simulink model "KugleArmTest1"  (R2018b)
settings: Solver=VariableStepAuto  StartTime=0.0  StopTime=100  RelTol=1e-3
libraries: vrlib x2, simulink x1, aerolibanimutils x1
settings Model: Creator=Yahya  LastModifiedBy=martinandersen

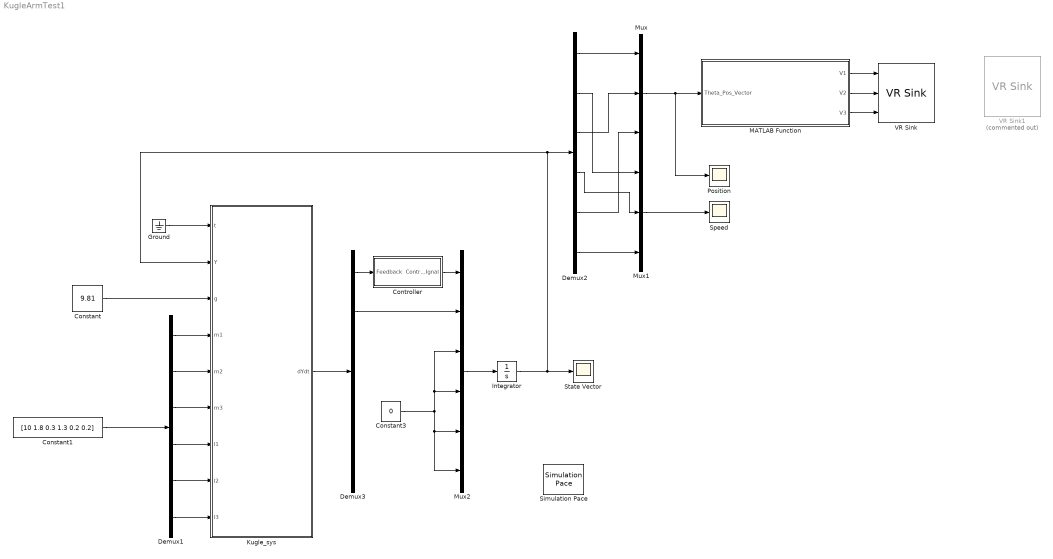
== system KugleArmTest1 ==
  Constant : Constant  Value=9.81
  Constant1 : Constant  Value=[10 1.8 0.3 1.3 0.2 0.2]
  Constant3 : Constant  Value=0
  Controller : Subsystem
  Demux1 : Demux  Outputs=6
  Demux2 : Demux  Outputs=6
  Demux3 : Demux  Outputs=6
  Ground : Ground
  Integrator : Integrator  InitialCondition=[1 0 90 0 45 0]*pi/180
  Kugle_sys : MATLAB Function  TreatAsAtomicUnit=on
  MATLAB Function : MATLAB Function  TreatAsAtomicUnit=on
  Mux : Mux  Inputs=3
  Mux1 : Mux  Inputs=3
  Mux2 : Mux  Inputs=6
  Position : Scope
  Simulation Pace : aerolibanimutils/Simulation Pace  SimulationPace=1  SleepMode=MATLAB Thread  OutputPaceError=off  SampleTime=1/30
      settings: AttributesFormatString=%<SimulationPace> sec/sec
  Speed : Scope
  State Vector : Scope
  VR Sink : vrlib/VR Sink  InstantiateOnLoad=on  SampleTime=0.1  ViewEnable=on  RemoteChange=off  RemoteView=off  FieldsWritten=JOINT_1.rotation.4.1.1.double#JOINT_2.rotation.4.1.1.double#JOINT_3.rotation.4.1.1.double  WorldFileName=Pendel3D1.wrl  AutoView=off  VideoDimensions=[]  AllowVariableSize=off  FigureProperties="{'Position', 'Name', 'Viewpoint', 'CameraBound', 'CameraDirection', 'CameraPosition', 'CameraUpVector', 'ZoomFactor', 'Antialiasing', 'Headlight', 'Lighting', 'NavPanel', 'Sound', 'StatusBar', 'Stereo3D', 'Stereo3DCameraOffset', 'Stereo3DHIT', 'ToolBar', 'Textures', 'Transparency', 'Triad', 'Wireframe', 'NavZones', 'NavMode', 'NavSpeed', 'CaptureFileFormat', 'CaptureFileName', 'Record2DCompressMethod', 'Record2DCompressQuality', 'Record2D', 'Record2DFileName', 'Record2DFPS'; [5.0000000000000000e+00   9.4000000000000000e+01   5.7600000000000000e+02   3.5000000000000000e+02], '', '', 'on', [0.0000000000000000e+00   0.0000000000000000e+00  -1.0000000000000000e+00], [0.0000000000000000e+00   0.0000000000000000e+00   1.0000000000000000e+01], [0.0000000000000000e+00   1.0000000000000000e+00   0.0000000000000000e+00], [1.0000000000000000e+00], 'on', 'on', 'on', 'halfbar', 'on', 'on', 'off', [1.0000000149011612e-01], [0.0000000000000000e+00], 'on', 'on', 'on', 'none', 'off', 'off', 'fly', 'normal', 'tif', '%f_anim_%n.tif', 'auto', [7.5000000000000000e+01], 'off', '%f_anim_%n.avi', 'auto'}"
      settings: SourceProductBaseCode=VR
  VR Sink1 : vrlib/VR Sink  Commented=on  InstantiateOnLoad=on  SampleTime=0.1  ViewEnable=on  RemoteChange=off  RemoteView=off  FieldsWritten=JOINT_1.rotation.4.1.1.double#JOINT_2.rotation.4.1.1.double#JOINT_3.rotation.4.1.1.double  WorldFileName=Pendel3D1.wrl  AutoView=off  VideoDimensions=[]  AllowVariableSize=off
      settings: SourceProductBaseCode=VR
  wires:
  Constant/1 -> Kugle_sys/3(g)
  Integrator/1 -> Kugle_sys/2(Y), Demux2/1, State Vector/1
  Ground/1 -> Kugle_sys/1(t)
  Demux1/1 -> Kugle_sys/4(m1)
  Demux1/2 -> Kugle_sys/5(m2)
  Demux1/3 -> Kugle_sys/6(m3)
  Demux1/4 -> Kugle_sys/7(l1)
  Demux1/5 -> Kugle_sys/8(l2)
  Demux1/6 -> Kugle_sys/9(l3)
  Constant1/1 -> Demux1/1
  Demux2/1 -> Mux/1
  Mux/1 -> MATLAB Function/1(Theta_Pos_Vector), Position/1
  Mux1/1 -> Speed/1
  Demux2/3 -> Mux/2
  Demux2/5 -> Mux/3
  Demux2/2 -> Mux1/1
  Demux2/4 -> Mux1/2
  Demux2/6 -> Mux1/3
  MATLAB Function/1(V1) -> VR Sink/1
  MATLAB Function/2(V2) -> VR Sink/2
  MATLAB Function/3(V3) -> VR Sink/3
  Kugle_sys/1(dYdt) -> Demux3/1
  Mux2/1 -> Integrator/1
  Constant3/1 -> Mux2/4, Mux2/3, Mux2/6, Mux2/5
  Demux3/2 -> Mux2/2
  Demux3/1 -> Controller/1(Feedback)
  Controller/1(Control SIgnal) -> Mux2/1

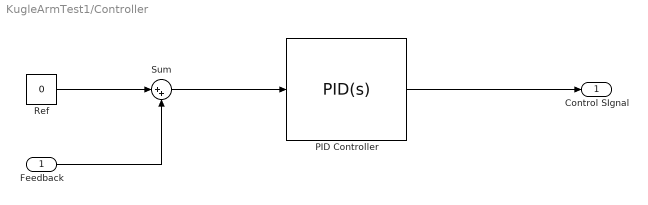
== system KugleArmTest1/Controller ==
  Feedback : Inport
  PID Controller : simulink/Continuous/PID Controller  Controller=PID  Form=Parallel  TimeDomain=Continuous-time  SampleTime=-1  IntegratorMethod=Forward Euler  FilterMethod=Forward Euler  ControllerParametersSource=internal  P=-0.0250583330761755  I=-0.00117310030702187  D=0  UseFilter=on  N=5.45397025421619  TunerSelectOption=Transfer Function Based (PID Tuner App)  InitialConditionSource=internal  InitialConditionForIntegrator=0  InitialConditionForFilter=0  DifferentiatorICPrevScaledInput=0  ExternalReset=none  TrackingMode=off  Kt=1  LimitOutput=off  UpperSaturationLimit=inf  LowerSaturationLimit=-inf  LinearizeAsGain=on  AntiWindupMode=none  Kb=1  POutMin=[]  POutMax=[]  IOutMin=[]  IOutMax=[]  DOutMin=[]  DOutMax=[]  NOutMin=[]  NOutMax=[]  SumOutMin=[]  SumOutMax=[]  SaturationOutMin=[]  SaturationOutMax=[]  PParamMin=[]  PParamMax=[]  IParamMin=[]  IParamMax=[]  DParamMin=[]  DParamMax=[]  NParamMin=[]  NParamMax=[]  KbParamMin=[]  KbParamMax=[]  KtParamMin=[]  KtParamMax=[]  KbOutMin=[]  KbOutMax=[]  KtOutMin=[]  KtOutMax=[]  IntegratorOutMin=[]  IntegratorOutMax=[]  FilterOutMin=[]  FilterOutMax=[]  SumI1OutMin=[]  SumI1OutMax=[]  SumI2OutMin=[]  SumI2OutMax=[]  SumI3OutMin=[]  SumI3OutMax=[]  SumI4OutMin=[]  SumI4OutMax=[]  SumDOutMin=[]  SumDOutMax=[]  DifferentiatorOutMin=[]  DifferentiatorOutMax=[]  FilterDiffOutCoefMin=[]  FilterDiffOutCoefMax=[]  ReciprocalOutMin=[]  ReciprocalOutMax=[]  SumDenOutMin=[]  SumDenOutMax=[]  SumNumOutMin=[]  SumNumOutMax=[]  DivideOutMin=[]  DivideOutMax=[]  IntegratorContinuousStateAttributes=''  IntegratorStateMustResolveToSignalObject=off  IntegratorRTWStateStorageClass=Auto  FilterContinuousStateAttributes=''  FilterStateMustResolveToSignalObject=off  FilterRTWStateStorageClass=Auto  ParallelPVariant=InternalParameters  IdealPVariant=Disabled  IVariant=InternalParameters  DVariant=InternalParameters  IntegratorVariant=Continuous  SatVariant=Disabled  AWVariant=Passthrough  PCopyVariant=Disabled  TRVariant=Disabled  FdbkBlocksVariant=Forward  IdealPFdbkVariant=Disabled  SatFdbkVariant=Disabled  DerivativeFilterVariant=ContFilter  NVariant=InternalParameters  NCopyVariant=Disabled  FilterICVariant=InternalICsFilter  IntegratorICVariant=InternalICs  ExternalResetVariant=Disabled  TRSumVariant=Passthrough  SumFdbkVariant=Disabled  SumVariant=Sum_PID
  Ref : Constant  Value=0
  Sum : Sum  Inputs=|++
  Control SIgnal : Outport
  wires:
  Ref/1 -> Sum/1
  Feedback/1 -> Sum/2
  Sum/1 -> PID Controller/1
  PID Controller/1 -> Control SIgnal/1

== matlab function KugleArmTest1/MATLAB Function ==
  data: Theta_Pos_Vector input; V1 output; V2 output; V3 output
function [V1, V2, V3] = AngleToRotationMatrix(Theta_Pos_Vector)

th1 = Theta_Pos_Vector(1);
th2 = Theta_Pos_Vector(2);
th3 = Theta_Pos_Vector(3);

V1 = [0 0 1 th1]';
V2 = [0 0 1 -th2]';
V3 = [0 0 1 -th3]';

== matlab function KugleArmTest1/Kugle_sys ==
  data: t input; dYdt output; Y input; g input; m1 input; m2 input; m3 input; l1 input; l2 input; l3 input
function dYdt = Kugle_sys(t,Y,g,m1,m2,m3,l1,l2,l3)
%#codegen

%    This function was generated by the Symbolic Math Toolbox version 8.2.
%    04-Apr-2019 11:38:35

t3 = Y(5);
t2 = cos(t3);
t4 = t2.^2;
t5 = m2.^2;
t6 = sin(t3);
t7 = m3.^2;
t8 = t6.^2;
t10 = Y(1);
t11 = Y(3);
t12 = t10-t11;
t9 = cos(t12);
t13 = t9.^2;
t14 = -t3+t10;
t15 = cos(t14);
t16 = -t3+t11;
t17 = cos(t16);
t18 = cos(t10);
t19 = cos(t11);
t20 = sin(t10);
t21 = sin(t11);
t22 = Y(4);
t23 = sin(t12);
t24 = t22.^2;
t25 = Y(6);
t26 = sin(t14);
t27 = t25.^2;
t28 = Y(2);
t29 = t28.^2;
t30 = sin(t16);
t31 = t21.^2;
t32 = t4.*t5;
t33 = t4.*t7;
t34 = t5.*t8;
t35 = t7.*t8;
t36 = m1.*m2.*t4;
t37 = m1.*m3.*t4;
t38 = m2.*m3.*t4.*2.0;
t39 = m1.*m2.*t8;
t40 = m1.*m3.*t8;
t41 = m2.*m3.*t8.*2.0;
t42 = t2.*t7.*t9.*t17.*t18;
t43 = t2.*t7.*t9.*t15.*t19;
t44 = t6.*t7.*t9.*t17.*t20;
t45 = t6.*t7.*t9.*t15.*t21;
t46 = m2.*m3.*t2.*t9.*t17.*t18;
t47 = m2.*m3.*t2.*t9.*t15.*t19;
t48 = m2.*m3.*t6.*t9.*t17.*t20;
t49 = m2.*m3.*t6.*t9.*t15.*t21;
t50 = t32+t33+t34+t35+t36+t37+t38+t39+t40+t41+t42+t43+t44+t45+t46+t47+t48+t49-t4.*t5.*t13-t4.*t7.*t13-t5.*t8.*t13-t7.*t8.*t13-m2.*m3.*t4.*t13.*2.0-m2.*m3.*t8.*t13.*2.0-t2.*t7.*t15.*t18-t2.*t7.*t17.*t19-t6.*t7.*t15.*t20-t6.*t7.*t17.*t21-m2.*m3.*t2.*t15.*t18-m1.*m3.*t2.*t17.*t19-m2.*m3.*t2.*t17.*t19-m2.*m3.*t6.*t15.*t20-m1.*m3.*t6.*t17.*t21-m2.*m3.*t6.*t17.*t21;
t51 = 1.0./t50;
t52 = t20.^2;
dYdt = [t28;-(t51.*(g.*t6.*t7.*t15-g.*t4.*t5.*t20-g.*t4.*t7.*t20-g.*t5.*t8.*t20-g.*t7.*t8.*t20+g.*m2.*m3.*t6.*t15-g.*m1.*m2.*t4.*t20-g.*m1.*m3.*t4.*t20-g.*m2.*m3.*t4.*t20.*2.0-g.*m1.*m2.*t8.*t20-g.*m1.*m3.*t8.*t20-g.*m2.*m3.*t8.*t20.*2.0+g.*t4.*t5.*t9.*t21-g.*t6.*t7.*t9.*t17+g.*t4.*t7.*t9.*t21+g.*t5.*t8.*t9.*t21+g.*t7.*t8.*t9.*t21-g.*t6.*t7.*t15.*t31+l2.*t4.*t5.*t23.*t24+l2.*t4.*t7.*t23.*t24+l2.*t5.*t8.*t23.*t24+l2.*t7.*t8.*t23.*t24+l3.*t4.*t7.*t26.*t27+l3.*t7.*t8.*t26.*t27+l2.*m2.*m3.*t4.*t23.*t24.*2.0+l2.*m2.*m3.*t8.*t23.*t24.*2.0+l3.*m2.*m3.*t4.*t26.*t27+l3.*m2.*m3.*t8.*t26.*t27-g.*t2.*t7.*t15.*t19.*t21+g.*t2.*t7.*t17.*t19.*t20+g.*t6.*t7.*t17.*t20.*t21+l1.*t4.*t5.*t9.*t23.*t29+l2.*t2.*t7.*t15.*t21.*t24+l1.*t4.*t7.*t9.*t23.*t29-l2.*t6.*t7.*t15.*t19.*t24+l1.*t2.*t7.*t15.*t20.*t29+l1.*t5.*t8.*t9.*t23.*t29-l1.*t6.*t7.*t15.*t18.*t29+l1.*t7.*t8.*t9.*t23.*t29-l3.*t4.*t7.*t9.*t27.*t30-l3.*t7.*t8.*t9.*t27.*t30-g.*m2.*m3.*t6.*t9.*t17+g.*m2.*m3.*t4.*t9.*t21.*2.0+g.*m2.*m3.*t8.*t9.*t21.*2.0-g.*m2.*m3.*t6.*t15.*t31+g.*m1.*m3.*t2.*t17.*t19.*t20-g.*m2.*m3.*t2.*t15.*t19.*t21+g.*m2.*m3.*t2.*t17.*t19.*t20+g.*m1.*m3.*t6.*t17.*t20.*t21+g.*m2.*m3.*t6.*t17.*t20.*t21+l2.*m2.*m3.*t2.*t15.*t21.*t24+l1.*m2.*m3.*t4.*t9.*t23.*t29.*2.0-l2.*m2.*m3.*t6.*t15.*t19.*t24+l1.*m2.*m3.*t2.*t15.*t20.*t29-l1.*m2.*m3.*t6.*t15.*t18.*t29+l1.*m2.*m3.*t8.*t9.*t23.*t29.*2.0-l3.*m2.*m3.*t4.*t9.*t27.*t30-l3.*m2.*m3.*t8.*t9.*t27.*t30-l2.*t2.*t7.*t9.*t17.*t21.*t24+l2.*t6.*t7.*t9.*t17.*t19.*t24-l1.*t2.*t7.*t9.*t17.*t20.*t29+l1.*t6.*t7.*t9.*t17.*t18.*t29-l2.*t2.*t7.*t17.*t19.*t23.*t24-l1.*t2.*t7.*t15.*t19.*t23.*t29-l2.*t6.*t7.*t17.*t21.*t23.*t24-l3.*t2.*t7.*t17.*t19.*t26.*t27-l1.*t6.*t7.*t15.*t21.*t23.*t29+l3.*t2.*t7.*t15.*t19.*t27.*t30-l3.*t6.*t7.*t17.*t21.*t26.*t27+l3.*t6.*t7.*t15.*t21.*t27.*t30-l2.*m2.*m3.*t2.*t9.*t17.*t21.*t24+l2.*m2.*m3.*t6.*t9.*t17.*t19.*t24-l1.*m2.*m3.*t2.*t9.*t17.*t20.*t29+l1.*m2.*m3.*t6.*t9.*t17.*t18.*t29-l2.*m2.*m3.*t2.*t17.*t19.*t23.*t24-l1.*m2.*m3.*t2.*t15.*t19.*t23.*t29-l2.*m2.*m3.*t6.*t17.*t21.*t23.*t24-l1.*m2.*m3.*t6.*t15.*t21.*t23.*t29))./l1;t22;(t51.*(g.*t4.*t5.*t21-g.*t6.*t7.*t17+g.*t4.*t7.*t21+g.*t5.*t8.*t21+g.*t7.*t8.*t21-g.*m1.*m3.*t6.*t17+g.*m1.*m2.*t4.*t21-g.*m2.*m3.*t6.*t17+g.*m1.*m3.*t4.*t21+g.*m2.*m3.*t4.*t21.*2.0+g.*m1.*m2.*t8.*t21+g.*m1.*m3.*t8.*t21+g.*m2.*m3.*t8.*t21.*2.0+g.*t6.*t7.*t9.*t15-g.*t4.*t5.*t9.*t20-g.*t4.*t7.*t9.*t20-g.*t5.*t8.*t9.*t20-g.*t7.*t8.*t9.*t20+g.*t6.*t7.*t17.*t52+l1.*t4.*t5.*t23.*t29+l1.*t4.*t7.*t23.*t29+l1.*t5.*t8.*t23.*t29+l1.*t7.*t8.*t23.*t29-l3.*t4.*t7.*t27.*t30-l3.*t7.*t8.*t27.*t30+l1.*m1.*m2.*t4.*t23.*t29+l1.*m1.*m3.*t4.*t23.*t29+l1.*m2.*m3.*t4.*t23.*t29.*2.0+l1.*m1.*m2.*t8.*t23.*t29+l1.*m1.*m3.*t8.*t23.*t29+l1.*m2.*m3.*t8.*t23.*t29.*2.0-l3.*m1.*m3.*t4.*t27.*t30-l3.*m2.*m3.*t4.*t27.*t30-l3.*m1.*m3.*t8.*t27.*t30-l3.*m2.*m3.*t8.*t27.*t30-g.*t2.*t7.*t15.*t18.*t21+g.*t2.*t7.*t17.*t18.*t20-g.*t6.*t7.*t15.*t20.*t21+l2.*t4.*t5.*t9.*t23.*t24+l2.*t4.*t7.*t9.*t23.*t24+l2.*t5.*t8.*t9.*t23.*t24-l2.*t2.*t7.*t17.*t21.*t24+l2.*t7.*t8.*t9.*t23.*t24+l2.*t6.*t7.*t17.*t19.*t24-l1.*t2.*t7.*t17.*t20.*t29+l3.*t4.*t7.*t9.*t26.*t27+l1.*t6.*t7.*t17.*t18.*t29+l3.*t7.*t8.*t9.*t26.*t27+g.*m2.*m3.*t6.*t9.*t15-g.*m1.*m2.*t4.*t9.*t20-g.*m1.*m3.*t4.*t9.*t20-g.*m2.*m3.*t4.*t9.*t20.*2.0-g.*m1.*m2.*t8.*t9.*t20-g.*m1.*m3.*t8.*t9.*t20-g.*m2.*m3.*t8.*t9.*t20.*2.0+g.*m1.*m3.*t6.*t17.*t52+g.*m2.*m3.*t6.*t17.*t52+g.*m1.*m3.*t2.*t17.*t18.*t20-g.*m2.*m3.*t2.*t15.*t18.*t21+g.*m2.*m3.*t2.*t17.*t18.*t20-g.*m2.*m3.*t6.*t15.*t20.*t21+l2.*m2.*m3.*t4.*t9.*t23.*t24.*2.0-l2.*m1.*m3.*t2.*t17.*t21.*t24-l2.*m2.*m3.*t2.*t17.*t21.*t24+l2.*m2.*m3.*t8.*t9.*t23.*t24.*2.0+l2.*m1.*m3.*t6.*t17.*t19.*t24-l1.*m1.*m3.*t2.*t17.*t20.*t29+l2.*m2.*m3.*t6.*t17.*t19.*t24-l1.*m2.*m3.*t2.*t17.*t20.*t29+l3.*m2.*m3.*t4.*t9.*t26.*t27+l1.*m1.*m3.*t6.*t17.*t18.*t29+l1.*m2.*m3.*t6.*t17.*t18.*t29+l3.*m2.*m3.*t8.*t9.*t26.*t27+l2.*t2.*t7.*t9.*t15.*t21.*t24-l2.*t6.*t7.*t9.*t15.*t19.*t24+l1.*t2.*t7.*t9.*t15.*t20.*t29-l1.*t6.*t7.*t9.*t15.*t18.*t29-l2.*t2.*t7.*t17.*t18.*t23.*t24-l1.*t2.*t7.*t15.*t18.*t23.*t29-l2.*t6.*t7.*t17.*t20.*t23.*t24-l3.*t2.*t7.*t17.*t18.*t26.*t27-l1.*t6.*t7.*t15.*t20.*t23.*t29+l3.*t2.*t7.*t15.*t18.*t27.*t30-l3.*t6.*t7.*t17.*t20.*t26.*t27+l3.*t6.*t7.*t15.*t20.*t27.*t30+l2.*m2.*m3.*t2.*t9.*t15.*t21.*t24-l2.*m2.*m3.*t6.*t9.*t15.*t19.*t24+l1.*m2.*m3.*t2.*t9.*t15.*t20.*t29-l1.*m2.*m3.*t6.*t9.*t15.*t18.*t29-l2.*m2.*m3.*t2.*t17.*t18.*t23.*t24-l1.*m2.*m3.*t2.*t15.*t18.*t23.*t29-l2.*m2.*m3.*t6.*t17.*t20.*t23.*t24-l1.*m2.*m3.*t6.*t15.*t20.*t23.*t29))./l2;t25;-(-g.*t5.*t6-g.*t6.*t7-g.*m1.*m2.*t6-g.*m1.*m3.*t6-g.*m2.*m3.*t6.*2.0+g.*t5.*t6.*t13+g.*t6.*t7.*t13+g.*t5.*t6.*t31+g.*t6.*t7.*t31+g.*t5.*t6.*t52+g.*t6.*t7.*t52+g.*m2.*m3.*t6.*t13.*2.0+g.*m1.*m2.*t6.*t31+g.*m1.*m3.*t6.*t31+g.*m2.*m3.*t6.*t31.*2.0+g.*m1.*m2.*t6.*t52+g.*m1.*m3.*t6.*t52+g.*m2.*m3.*t6.*t52.*2.0+g.*t2.*t5.*t18.*t20+g.*t2.*t5.*t19.*t21+g.*t2.*t7.*t18.*t20+g.*t2.*t7.*t19.*t21-l2.*t2.*t5.*t21.*t24-l2.*t2.*t7.*t21.*t24+l2.*t5.*t6.*t19.*t24-l1.*t2.*t5.*t20.*t29+l2.*t6.*t7.*t19.*t24-l1.*t2.*t7.*t20.*t29+l1.*t5.*t6.*t18.*t29+l1.*t6.*t7.*t18.*t29-l2.*m1.*m2.*t2.*t21.*t24-l2.*m1.*m3.*t2.*t21.*t24+l2.*m1.*m2.*t6.*t19.*t24-l2.*m2.*m3.*t2.*t21.*t24.*2.0-l1.*m1.*m2.*t2.*t20.*t29+l2.*m1.*m3.*t6.*t19.*t24-l1.*m1.*m3.*t2.*t20.*t29+l2.*m2.*m3.*t6.*t19.*t24.*2.0+l1.*m1.*m2.*t6.*t18.*t29-l1.*m2.*m3.*t2.*t20.*t29.*2.0+l1.*m1.*m3.*t6.*t18.*t29+l1.*m2.*m3.*t6.*t18.*t29.*2.0-g.*t2.*t5.*t9.*t18.*t21-g.*t2.*t5.*t9.*t19.*t20-g.*t2.*t7.*t9.*t18.*t21-g.*t2.*t7.*t9.*t19.*t20-g.*t5.*t6.*t9.*t20.*t21.*2.0-g.*t6.*t7.*t9.*t20.*t21.*2.0+l2.*t2.*t5.*t13.*t21.*t24+l2.*t2.*t7.*t13.*t21.*t24-l2.*t5.*t6.*t13.*t19.*t24+l1.*t2.*t5.*t13.*t20.*t29-l2.*t6.*t7.*t13.*t19.*t24+l1.*t2.*t7.*t13.*t20.*t29-l1.*t5.*t6.*t13.*t18.*t29-l1.*t6.*t7.*t13.*t18.*t29-l2.*t2.*t5.*t18.*t23.*t24-l2.*t2.*t7.*t18.*t23.*t24+l1.*t2.*t5.*t19.*t23.*t29-l2.*t5.*t6.*t20.*t23.*t24+l1.*t2.*t7.*t19.*t23.*t29-l2.*t6.*t7.*t20.*t23.*t24-l3.*t2.*t7.*t18.*t26.*t27+l1.*t5.*t6.*t21.*t23.*t29+l1.*t6.*t7.*t21.*t23.*t29-l3.*t2.*t7.*t19.*t27.*t30-l3.*t6.*t7.*t20.*t26.*t27-l3.*t6.*t7.*t21.*t27.*t30+g.*m1.*m2.*t2.*t18.*t20+g.*m1.*m3.*t2.*t18.*t20+g.*m1.*m2.*t2.*t19.*t21+g.*m2.*m3.*t2.*t18.*t20.*2.0+g.*m1.*m3.*t2.*t19.*t21+g.*m2.*m3.*t2.*t19.*t21.*2.0-g.*m1.*m2.*t2.*t9.*t19.*t20-g.*m1.*m3.*t2.*t9.*t19.*t20-g.*m2.*m3.*t2.*t9.*t18.*t21.*2.0-g.*m2.*m3.*t2.*t9.*t19.*t20.*2.0-g.*m1.*m2.*t6.*t9.*t20.*t21-g.*m1.*m3.*t6.*t9.*t20.*t21-g.*m2.*m3.*t6.*t9.*t20.*t21.*4.0+l2.*m2.*m3.*t2.*t13.*t21.*t24.*2.0-l2.*m2.*m3.*t6.*t13.*t19.*t24.*2.0+l1.*m2.*m3.*t2.*t13.*t20.*t29.*2.0-l1.*m2.*m3.*t6.*t13.*t18.*t29.*2.0-l2.*m2.*m3.*t2.*t18.*t23.*t24.*2.0+l1.*m1.*m2.*t2.*t19.*t23.*t29+l1.*m1.*m3.*t2.*t19.*t23.*t29+l1.*m2.*m3.*t2.*t19.*t23.*t29.*2.0-l2.*m2.*m3.*t6.*t20.*t23.*t24.*2.0-l3.*m2.*m3.*t2.*t18.*t26.*t27+l1.*m1.*m2.*t6.*t21.*t23.*t29+l1.*m1.*m3.*t6.*t21.*t23.*t29+l1.*m2.*m3.*t6.*t21.*t23.*t29.*2.0-l3.*m1.*m3.*t2.*t19.*t27.*t30-l3.*m2.*m3.*t2.*t19.*t27.*t30-l3.*m2.*m3.*t6.*t20.*t26.*t27-l3.*m1.*m3.*t6.*t21.*t27.*t30-l3.*m2.*m3.*t6.*t21.*t27.*t30+l2.*t2.*t5.*t9.*t19.*t23.*t24+l2.*t2.*t7.*t9.*t19.*t23.*t24-l1.*t2.*t5.*t9.*t18.*t23.*t29-l1.*t2.*t7.*t9.*t18.*t23.*t29+l2.*t5.*t6.*t9.*t21.*t23.*t24+l2.*t6.*t7.*t9.*t21.*t23.*t24-l1.*t5.*t6.*t9.*t20.*t23.*t29+l3.*t2.*t7.*t9.*t19.*t26.*t27-l1.*t6.*t7.*t9.*t20.*t23.*t29+l3.*t2.*t7.*t9.*t18.*t27.*t30+l3.*t6.*t7.*t9.*t21.*t26.*t27+l3.*t6.*t7.*t9.*t20.*t27.*t30+l2.*m2.*m3.*t2.*t9.*t19.*t23.*t24.*2.0-l1.*m2.*m3.*t2.*t9.*t18.*t23.*t29.*2.0+l2.*m2.*m3.*t6.*t9.*t21.*t23.*t24.*2.0+l3.*m2.*m3.*t2.*t9.*t19.*t26.*t27-l1.*m2.*m3.*t6.*t9.*t20.*t23.*t29.*2.0+l3.*m2.*m3.*t2.*t9.*t18.*t27.*t30+l3.*m2.*m3.*t6.*t9.*t21.*t26.*t27+l3.*m2.*m3.*t6.*t9.*t20.*t27.*t30)./(l3.*t4.*t5+l3.*t4.*t7+l3.*t5.*t8+l3.*t7.*t8+l3.*m1.*m2.*t4+l3.*m1.*m3.*t4+l3.*m2.*m3.*t4.*2.0+l3.*m1.*m2.*t8+l3.*m1.*m3.*t8+l3.*m2.*m3.*t8.*2.0-l3.*t4.*t5.*t13-l3.*t4.*t7.*t13-l3.*t5.*t8.*t13-l3.*t7.*t8.*t13-l3.*m2.*m3.*t4.*t13.*2.0-l3.*m2.*m3.*t8.*t13.*2.0-l3.*t2.*t7.*t15.*t18-l3.*t2.*t7.*t17.*t19-l3.*t6.*t7.*t15.*t20-l3.*t6.*t7.*t17.*t21-l3.*m2.*m3.*t2.*t15.*t18-l3.*m1.*m3.*t2.*t17.*t19-l3.*m2.*m3.*t2.*t17.*t19-l3.*m2.*m3.*t6.*t15.*t20-l3.*m1.*m3.*t6.*t17.*t21-l3.*m2.*m3.*t6.*t17.*t21+l3.*t2.*t7.*t9.*t15.*t19+l3.*t2.*t7.*t9.*t17.*t18+l3.*t6.*t7.*t9.*t15.*t21+l3.*t6.*t7.*t9.*t17.*t20+l3.*m2.*m3.*t2.*t9.*t15.*t19+l3.*m2.*m3.*t2.*t9.*t17.*t18+l3.*m2.*m3.*t6.*t9.*t15.*t21+l3.*m2.*m3.*t6.*t9.*t17.*t20)];
